simulink model "digital_modulation"  (R2019b)
settings: Solver=VariableStepAuto  StartTime=0.0  StopTime=10.0  RelTol=1e-3
libraries: dsparch4 x4, commutil2 x4, dspsigops x3, commsink2 x2, commfilt2 x2, commrandsrc3 x2, dspquant2 x2
settings Model: Creator=DELL  LastModifiedBy=DELL

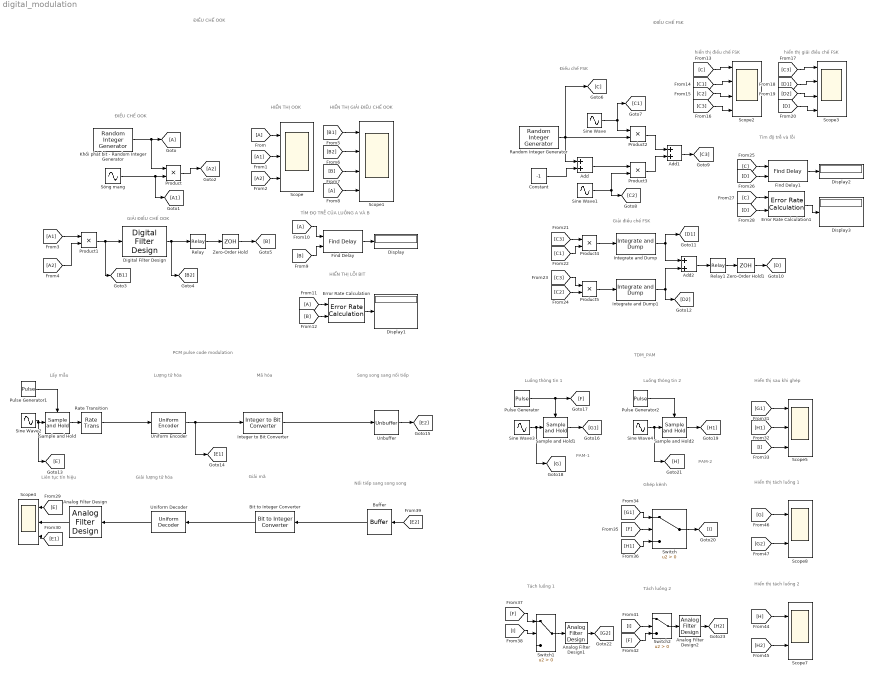
== system digital_modulation ==
  note: PAM-1
  note: HIỂN THỊ OOK
  note: ĐIỀU CHẾ OOK
  note: GIẢI ĐIỀU CHẾ OOK
  note: HIỂN THỊ GIẢI ĐIỀU CHẾ OOK
  note: TÌM ĐỌ TRỄ CỦA LUỒNG A VÀ B
  note: HIỂN THỊ LỖI BIT
  note: ĐIỀU CHẾ OOK
  note: hiển thị giải điều chế FSK
  note: ĐIỀU CHẾ FSK
  note: hiển thị điều chế FSK
  note: Giải điều chế FSK
  note: Điều chế FSK
  note: Tìm độ trễ và lỗi
  note: Lượng tử hóa
  note: Lấy mẫu
  note: Mã hóa
  note: Nối tiếp sang
      | song song
  note: Song song sang
      | nối tiếp
  note: Giải mã
  note: Giải lượng tử hóa
  note: Liên tục tín hiệu
  note: PCM pulse code modulation
  note: Luồng thông tin 1
  note: Luồng thông tin 2
  note: Ghép kênh
  note: Hiển thị sau khi ghép
  note: PAM-2
  note: Tách luồng 1
  note: Tách luồng 2
  note: Hiển thị tách luồng 2
  note: Hiển thị tách luồng 1
  note: TDM_PAM
  Add : Sum
  Add1 : Sum
  Add2 : Sum
  Analog Filter Design : dsparch4/Analog Filter Design  method=Butterworth  filttype=Lowpass  N=12  Wlo=2*pi*4000  Whi=80  Rp=2  Rs=40
  Analog Filter Design1 : dsparch4/Analog Filter Design  method=Butterworth  filttype=Lowpass  N=12  Wlo=2*pi*2500  Whi=80  Rp=2  Rs=40
  Analog Filter Design2 : dsparch4/Analog Filter Design  method=Butterworth  filttype=Lowpass  N=12  Wlo=2*pi*1500  Whi=80  Rp=2  Rs=40
  Bit to Integer Converter : commutil2/Bit to Integer Converter  nbits=3  bitOrder=MSB first  signedOutputValues=Unsigned  outDtype=Inherit via internal rule  outDtypeSigned=Inherit via internal rule
      settings: SourceProductName=Communications Toolbox
  Buffer : Buffer  N=3  OutputFrames=off
  Constant : Constant  Value=-1
  Digital Filter Design : dsparch4/Digital Filter Design  mwdsp_browser_bugfix_var=off
  Display{,1..3} (4 alike) : Display
  Error Rate Calculation : commsink2/Error Rate Calculation  N=1  st_delay=0  cp_mode=Entire frame  subframe=[]  PMode=Port  WsName=ErrorVec  RsMode2=off  stop=off  numErr=100  maxBits=1e6
      settings: SourceProductName=Communications Toolbox
  Error Rate Calculation1 : commsink2/Error Rate Calculation  N=1  st_delay=0  cp_mode=Entire frame  subframe=[]  PMode=Port  WsName=ErrorVec  RsMode2=off  stop=off  numErr=100  maxBits=1e6
      settings: SourceProductName=Communications Toolbox
  Find Delay : commutil2/Find Delay  corrLength=200  chgSigOP=off  stopUpdate=off  numConstDelay=3
      settings: SourceProductName=Communications Toolbox  SourceProductBaseCode=CM
  Find Delay1 : commutil2/Find Delay  corrLength=200  chgSigOP=off  stopUpdate=off  numConstDelay=3
      settings: SourceProductName=Communications Toolbox  SourceProductBaseCode=CM
  Integer to Bit Converter : commutil2/Integer to Bit Converter  nbits=3  signedInputValues=Unsigned  bitOrder=MSB first  outDtype=Inherit via internal rule
      settings: SourceProductName=Communications Toolbox
  Integrate and Dump : commfilt2/Integrate and Dump  obssamples=100  offsetsamples=0  nodump=off  roundingMode=Floor  overflowMode=off  outputDataTypeStr=Inherit: Same as accumulator  outputLastDataTypeStr=Inherit: Same as accumulator
      settings: SourceProductName=Communications Toolbox
  Integrate and Dump1 : commfilt2/Integrate and Dump  obssamples=100  offsetsamples=0  nodump=off  roundingMode=Floor  overflowMode=off  outputDataTypeStr=Inherit: Same as accumulator  outputLastDataTypeStr=Inherit: Same as accumulator
      settings: SourceProductName=Communications Toolbox
  Khối phát bit - Random Integer Generator : commrandsrc3/Random Integer Generator  SetSize=2  SeedSource=Auto  Seed=0  SampleTime=1/1000  SamplesPerFrame=1  OutputDataType=double  SimulateUsing=Interpreted execution
      settings: SourceProductName=Communications Toolbox
  Product{,1..5} (6 alike) : Product
  Pulse Generator : DiscretePulseGenerator  PulseType=Time based  Period=1/8000  PulseWidth=5
  Pulse Generator1 : DiscretePulseGenerator  PulseType=Time based  Period=1/8000  PulseWidth=5
  Pulse Generator2 : DiscretePulseGenerator  PulseType=Time based  Period=1/8000  PulseWidth=5
  Random Integer Generator : commrandsrc3/Random Integer Generator  SetSize=2  SeedSource=Parameter  Seed=0  SampleTime=1/1000  SamplesPerFrame=1  OutputDataType=double  SimulateUsing=Interpreted execution
      settings: SourceProductName=Communications Toolbox
  Rate Transition : RateTransition  OutPortSampleTime=1/8000
  Relay : Relay  OnSwitchValue=0.25  OffSwitchValue=0.25
  Relay1 : Relay  OnSwitchValue=0  OffSwitchValue=0
  Sample and Hold : dspsigops/Sample and Hold  trig=Rising edge  initCond=0  latchinput=off
  Sample and Hold1 : dspsigops/Sample and Hold  trig=Rising edge  initCond=0  latchinput=off
  Sample and Hold2 : dspsigops/Sample and Hold  trig=Rising edge  initCond=0  latchinput=off
  Scope : Scope  NumInputPorts=3
  Scope1 : Scope  NumInputPorts=4
  Scope2 : Scope  NumInputPorts=4
  Scope3 : Scope  NumInputPorts=4
  Scope4 : Scope  NumInputPorts=3
  Scope5 : Scope  NumInputPorts=3
  Scope7 : Scope  NumInputPorts=2
  Scope8 : Scope  NumInputPorts=2
  Sine Wave : Sin  Frequency=2*pi*10000  SampleTime=1/100000
  Sine Wave1 : Sin  Frequency=2*pi*11000  SampleTime=1/100000
  Sine Wave2 : Sin  Frequency=2*pi*3000  SampleTime=1/100000
  Sine Wave3 : Sin  Frequency=2*pi*2000  SampleTime=1/64000
  Sine Wave4 : Sin  Frequency=2*pi*1000  SampleTime=1/64000
  Switch : Switch  Criteria=u2 > Threshold
  Switch1 : Switch  Criteria=u2 > Threshold
  Switch2 : Switch  Criteria=u2 > Threshold
  Sóng mang : Sin  Frequency=2*pi*10000  SampleTime=1/100000
  Unbuffer : Unbuffer
  Uniform Decoder : dspquant2/Uniform Decoder  peak=1  bits=3  overflowMode=Saturate  otype=Double
      settings: SourceProductName=DSP System Toolbox  SourceProductBaseCode=DS
  Uniform Encoder : dspquant2/Uniform Encoder  peak=1  bits=3  otype=Unsigned integer
      settings: SourceProductName=DSP System Toolbox
  Zero-Order Hold : ZeroOrderHold  SampleTime=1/1000
  Zero-Order Hold1 : ZeroOrderHold  SampleTime=1/1000
  wires:
  Sóng mang/1 -> [A1], Product/2
  Khối phát bit - Random Integer Generator/1 -> [A], Product/1
  Product/1 -> [A2]
  [A] -> Scope/1
  [A1] -> Scope/2
  [A2] -> Scope/3
  Product1/1 -> [B1], Digital Filter Design/1
  [A1] -> Product1/1
  [A2] -> Product1/2
  Digital Filter Design/1 -> [B2], Relay/1
  Relay/1 -> Zero-Order Hold/1
  Zero-Order Hold/1 -> [B]
  [A] -> Scope1/4
  [B] -> Scope1/3
  [B2] -> Scope1/2
  [B1] -> Scope1/1
  Find Delay/1 -> Display/1
  [B] -> Find Delay/2
  [A] -> Find Delay/1
  [A] -> Error Rate Calculation/1
  [B] -> Error Rate Calculation/2
  Error Rate Calculation/1 -> Display1/1
  Random Integer Generator/1 -> [C], Add/1, Product2/2
  Constant/1 -> Add/2
  Sine Wave/1 -> [C1], Product2/1
  Add/1 -> Product3/1
  Sine Wave1/1 -> [C2], Product3/2
  Product2/1 -> Add1/1
  Product3/1 -> Add1/2
  Add1/1 -> [C3]
  [C] -> Scope2/1
  [C1] -> Scope2/2
  [C2] -> Scope2/3
  [C3] -> Scope2/4
  [D2] -> Scope3/3
  [C3] -> Scope3/1
  [D] -> Scope3/4
  [D1] -> Scope3/2
  [C3] -> Product4/1
  [C1] -> Product4/2
  [C2] -> Product5/2
  [C3] -> Product5/1
  Product4/1 -> Integrate and Dump/1
  Product5/1 -> Integrate and Dump1/1
  Integrate and Dump/1 -> [D1], Add2/1
  Integrate and Dump1/1 -> [D2], Add2/2
  Add2/1 -> Relay1/1
  Relay1/1 -> Zero-Order Hold1/1
  Zero-Order Hold1/1 -> [D]
  [C] -> Find Delay1/1
  [D] -> Find Delay1/2
  [C] -> Error Rate Calculation1/1
  [D] -> Error Rate Calculation1/2
  Find Delay1/1 -> Display2/1
  Error Rate Calculation1/1 -> Display3/1
  Sine Wave2/1 -> [E], Sample and Hold/1
  Pulse Generator1/1 -> Sample and Hold/Trigger
  Sample and Hold/1 -> Rate Transition/1
  Rate Transition/1 -> Uniform Encoder/1
  Uniform Encoder/1 -> [E1], Integer to Bit Converter/1
  Integer to Bit Converter/1 -> Unbuffer/1
  Unbuffer/1 -> [E2]
  Bit to Integer Converter/1 -> Uniform Decoder/1
  Buffer/1 -> Bit to Integer Converter/1
  Uniform Decoder/1 -> Analog Filter Design/1
  Analog Filter Design/1 -> Scope4/2
  [E] -> Scope4/1
  [E1] -> Scope4/3
  Sine Wave3/1 -> [G], Sample and Hold1/1
  Pulse Generator/1 -> [F], Sample and Hold1/Trigger
  Sample and Hold1/1 -> [G1]
  Sample and Hold2/1 -> [H1]
  Pulse Generator2/1 -> Sample and Hold2/Trigger
  Sine Wave4/1 -> Sample and Hold2/1, [H]
  [G1] -> Scope5/1
  [H1] -> Scope5/2
  [I] -> Scope5/3
  [G1] -> Switch/1
  [F] -> Switch/2
  [H1] -> Switch/3
  Switch/1 -> [I]
  [I] -> Switch1/2
  [F] -> Switch1/1
  [I] -> Switch2/2
  [F] -> Switch2/3
  Switch1/1 -> Analog Filter Design1/1
  Analog Filter Design1/1 -> [G2]
  Analog Filter Design2/1 -> [H2]
  Switch2/1 -> Analog Filter Design2/1
  [H] -> Scope7/1
  [H2] -> Scope7/2
  [G2] -> Scope8/2
  [G] -> Scope8/1
  [E2] -> Buffer/1
